simulink model "ROSCO_vs_ESC"  (R2025b)
settings: Solver=VariableStepAuto  StartTime=0.0  StopTime=4000  RelTol=1e-3
undefined symbols (not defined in the file): J, K_tau, ki_tau, kp_tau, lambda_opt, Ng, omega_g_min, omega_g_rated, R, tau_g_rated
libraries: simulink x1
settings Model: Creator=Administrator  LastModifiedBy=Administrator
settings DataIOCC: ReturnWorkspaceOutputs=off

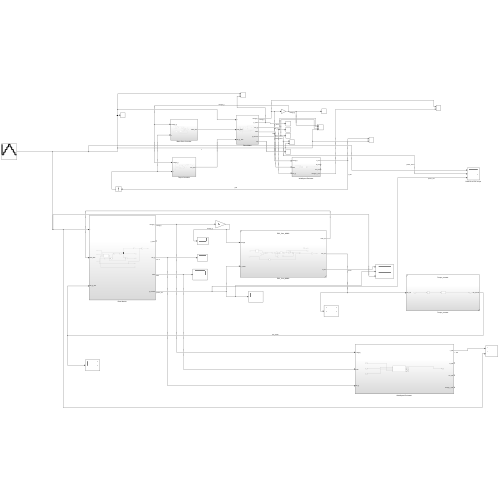
[thumbnail: Simulink's stored preview of the top-level diagram]
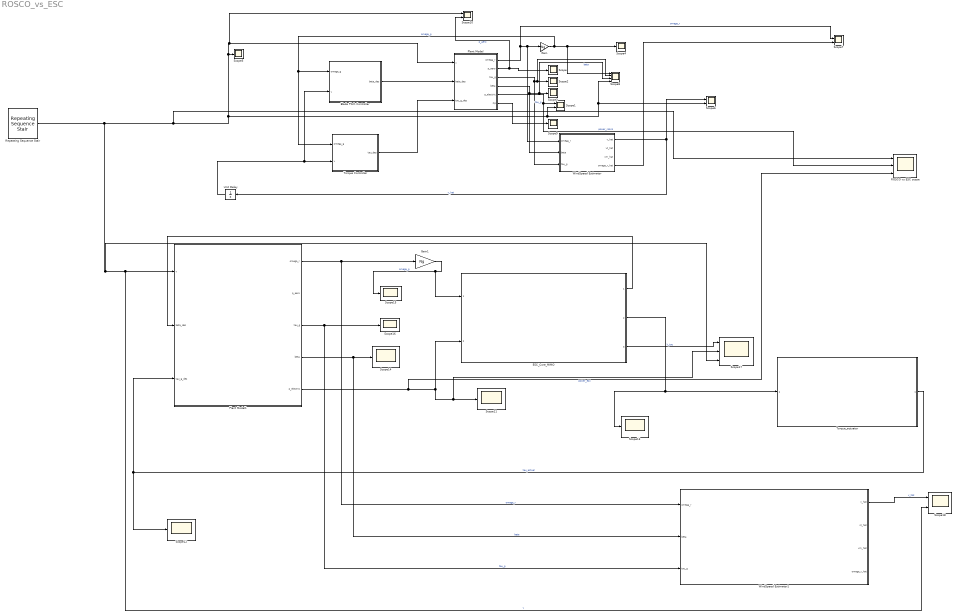
== system ROSCO_vs_ESC ==
  Blade Pitch Controller : Subsystem
  ESC_Core_MIMO : Subsystem  ReferencedSubsystem=ESC_Core_MIMO
  Gain : Gain  Gain=Ng
  Gain1 : Gain  Gain=Ng
  Plant Model : Subsystem
  Plant Model1 : Subsystem
  ROSCO vs ESC scope : Scope  NumInputPorts=3
      settings: ActiveDisplayYMinimum=5.5  ActiveDisplayYMaximum=10.5  DataLoggingVariableName=velData
  Repeating Sequence Stair : simulink/Sources/Repeating Sequence Stair  OutValues=[6 7 8 9 10 9 8 7 6]  tsamp=400  OutMin=[]  OutMax=[]  OutDataTypeStr=double  OutputDataTypeScalingMode=double  OutDataType=fixdt(0,8)  ConRadixGroup=Best Precision: Vector-wise  OutScaling=2^-12
  Scope{,2..5,9,11..16} (12 alike) : Scope
      Scope settings: ActiveDisplayYMinimum=-2.4283893779933713E+6  ActiveDisplayYMaximum=1.2562737180596253E+7  DataLoggingVariableName=ScopeData17
      Scope11 settings: ActiveDisplayYMinimum=-206726.94893270766  ActiveDisplayYMaximum=1.8605425403943695E+6  DataLoggingVariableName=ScopeData24
      Scope12 settings: ActiveDisplayYMinimum=25883.443415286834  ActiveDisplayYMaximum=45883.443415286834  DataLoggingVariableName=ScopeData25
      Scope13 settings: ActiveDisplayYMinimum=-6959.4378100502436  ActiveDisplayYMaximum=51916.667459968325  DataLoggingVariableName=ScopeData26
      Scope14 settings: ActiveDisplayYMinimum=-0.028992577845199295  ActiveDisplayYMaximum=0.2609332006067937  DataLoggingVariableName=ScopeData27
      Scope15 settings: ActiveDisplayYMinimum=5.9360506198945675  ActiveDisplayYMaximum=140.57554442094894  DataLoggingVariableName=ScopeData28
      Scope16 settings: ActiveDisplayYMinimum=-1  ActiveDisplayYMaximum=1  DataLoggingVariableName=ScopeData29
      Scope2 settings: ActiveDisplayYMinimum=-1  ActiveDisplayYMaximum=1  DataLoggingVariableName=ScopeData19
      Scope3 settings: ActiveDisplayYMinimum=-5.1281576222926013  ActiveDisplayYMaximum=18.391881826207097  DataLoggingVariableName=ScopeData4
      Scope4 settings: ActiveDisplayYMinimum=-16.100769807351526  ActiveDisplayYMaximum=150.23183145512027  DataLoggingVariableName=ScopeData5
      Scope5 settings: ActiveDisplayYMinimum=-1.9549334631606692  ActiveDisplayYMaximum=17.594401168446026  DataLoggingVariableName=ScopeData20
      Scope9 settings: ActiveDisplayYMinimum=-1  ActiveDisplayYMaximum=1  DataLoggingVariableName=ScopeData8
  Scope{1,6..7,10,18} (5 alike) : Scope  NumInputPorts=2
      Scope1 settings: ActiveDisplayYMinimum=1  ActiveDisplayYMaximum=21  DataLoggingVariableName=ScopeData18
      Scope10 settings: ActiveDisplayYMinimum=-0.49921784144822823  ActiveDisplayYMaximum=25.750782158551765  DataLoggingVariableName=ScopeData16
      Scope18 settings: ActiveDisplayYMinimum=-1.2495467804496814  ActiveDisplayYMaximum=11.245921024047135  DataLoggingVariableName=ScopeData31
      Scope6 settings: ActiveDisplayYMinimum=-1  ActiveDisplayYMaximum=1  DataLoggingVariableName=ScopeData21
      Scope7 settings: ActiveDisplayYMinimum=0.05875  ActiveDisplayYMaximum=1.47128  DataLoggingVariableName=ScopeData22
  Scope17 : Scope  NumInputPorts=3
      settings: ActiveDisplayYMinimum=2.97179268816189  ActiveDisplayYMaximum=7.2893156949682956  DataLoggingVariableName=ScopeData30
  Scope8 : Scope  NumInputPorts=4
      settings: ActiveDisplayYMinimum=5.68642269301175  ActiveDisplayYMaximum=142.8221957628943  DataLoggingVariableName=ScopeData23
  Torque Controller : Subsystem
  Torque_actuator : Subsystem  ReferencedSubsystem=Torque_actuator
  Unit Delay : UnitDelay  SampleTime=0.01  HasFrameUpgradeWarning=on
  WindSpeed Estimator : Subsystem
  WindSpeed Estimator1 : Subsystem
  wires:
  Plant Model/3(tau_g) -> Scope8/2, Scope2/1, WindSpeed Estimator/3(tau_g)  "tau_g"
  WindSpeed Estimator/4(omega_r_hat) -> Scope7/2
  Repeating Sequence Stair/1 -> Scope17/3, Scope18/2, Plant Model1/1(v), ROSCO vs ESC scope/1, Scope5/1, Scope10/1, Plant Model/1(v), Scope1/2, Scope8/4, Scope6/2  "v"
  WindSpeed Estimator/1(v_hat) -> Unit Delay/1, Scope6/1  "v_hat"
  Unit Delay/1 -> Blade Pitch Controller/2(v), Torque Controller/2(v)
  Torque Controller/1(tau_des) -> Plant Model/3(tau_g_des)
  Plant Model/6(Cp) -> Scope9/1
  Plant Model/2(p_aero) -> Scope10/2, Scope/1  "p_aero"
  Blade Pitch Controller/1(beta_des) -> Plant Model/2(beta_des)
  Gain/1 -> Blade Pitch Controller/1(omega_g), Torque Controller/1(omega_g), Scope8/1, Scope4/1  "omega_g"
  Plant Model/1(omega_r) -> WindSpeed Estimator/1(omega_r), Gain/1, Scope7/1  "omega_r"
  Plant Model/4(beta) -> Scope8/3, Scope3/1, WindSpeed Estimator/2(beta)  "beta"
  Plant Model/5(p_electric) -> ROSCO vs ESC scope/2, Scope1/1  "power_rosco"
  Plant Model1/3(tau_g) -> WindSpeed Estimator1/3(tau_g), Scope16/1  "tau_g"
  Torque_actuator/1 -> Scope12/1, Plant Model1/3(tau_g_des)  "tau_actual"
  Plant Model1/1(omega_r) -> WindSpeed Estimator1/1(omega_r), Gain1/1  "omega_r"
  ESC_Core_MIMO/3 -> Scope17/1  "k_tau"
  Plant Model1/5(p_electric) -> ROSCO vs ESC scope/3, Scope17/2, Scope11/1, ESC_Core_MIMO/2  "power_esc"
  ESC_Core_MIMO/1 -> Plant Model1/2(beta_des)
  Plant Model1/4(beta) -> WindSpeed Estimator1/2(beta), Scope14/1  "beta"
  WindSpeed Estimator1/1(v_hat) -> Scope18/1  "v_hat"
  Gain1/1 -> Scope15/1, ESC_Core_MIMO/1  "omega_g"
  ESC_Core_MIMO/2 -> Torque_actuator/1, Scope13/1

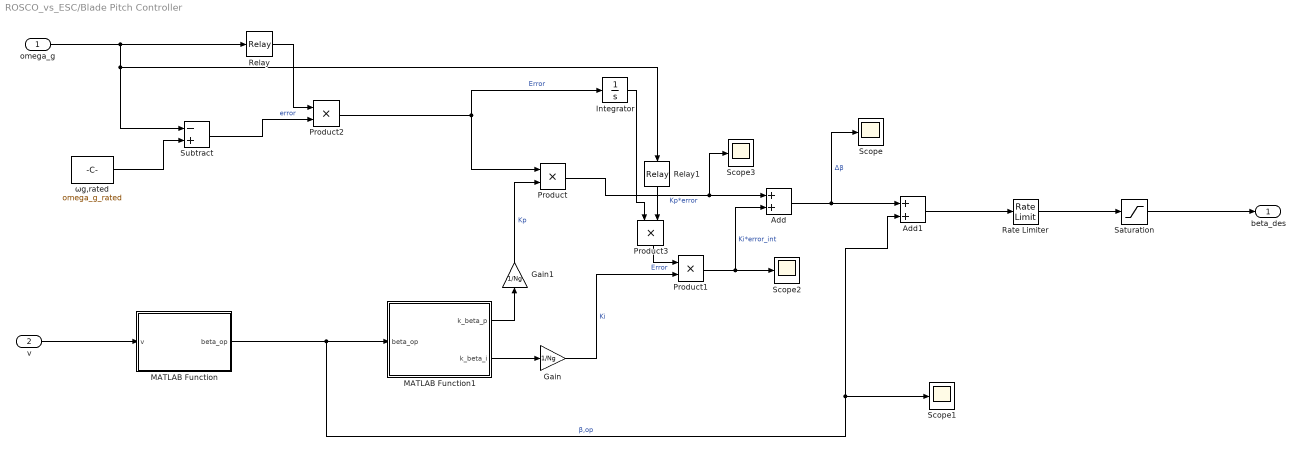
== system ROSCO_vs_ESC/Blade Pitch Controller ==
  omega_g : Inport
  v : Inport  Port=2
  Add : Sum
  Add1 : Sum
  Gain : Gain  Gain=1/Ng
  Gain1 : Gain  Gain=1/Ng
  Integrator : Integrator
  MATLAB Function : MATLAB Function  TreatAsAtomicUnit=on
  MATLAB Function1 : MATLAB Function  TreatAsAtomicUnit=on
  Product{,1..3} (4 alike) : Product
  Rate Limiter : RateLimiter  RisingSlewLimit=8  FallingSlewLimit=-8  SampleTimeMode=inherited
  Relay : Relay  OnSwitchValue=123.91  OffSwitchValue=121.91
  Relay1 : Relay  OnSwitchValue=123.91  OffSwitchValue=121.91
  Saturation : Saturate  UpperLimit=25  LowerLimit=0
  Scope{,1..3} (4 alike) : Scope
      Scope settings: ActiveDisplayYMinimum=-1  ActiveDisplayYMaximum=1  DataLoggingVariableName=ScopeData6
      Scope1 settings: ActiveDisplayYMinimum=-1  ActiveDisplayYMaximum=1  DataLoggingVariableName=ScopeData7
      Scope2 settings: ActiveDisplayYMinimum=-1  ActiveDisplayYMaximum=1  DataLoggingVariableName=ScopeData14
      Scope3 settings: ActiveDisplayYMinimum=-1  ActiveDisplayYMaximum=1  DataLoggingVariableName=ScopeData15
  Subtract : Sum  Inputs=-+
  ωg,rated : Constant  Value=omega_g_rated
  beta_des : Outport
  wires:
  Product1/1 -> Scope2/1, Add/2  "Ki*error_int"
  Add/1 -> Scope/1, Add1/1  "Δβ"
  MATLAB Function1/2(k_beta_i) -> Gain/1
  MATLAB Function/1(beta_op) -> Scope1/1, Add1/2, MATLAB Function1/1(beta_op)  "β,op"
  Product/1 -> Scope3/1, Add/1  "Kp*error"
  v/1 -> MATLAB Function/1(v)
  MATLAB Function1/1(k_beta_p) -> Gain1/1
  omega_g/1 -> Subtract/1, Relay1/1, Relay/1
  ωg,rated/1 -> Subtract/2
  Gain/1 -> Product1/2  "Ki"
  Gain1/1 -> Product/2  "Kp"
  Relay/1 -> Product2/1
  Subtract/1 -> Product2/2  "error"
  Product2/1 -> Integrator/1, Product/1  "Error"
  Rate Limiter/1 -> Saturation/1
  Saturation/1 -> beta_des/1
  Add1/1 -> Rate Limiter/1
  Relay1/1 -> Product3/2
  Integrator/1 -> Product3/1
  Product3/1 -> Product1/1  "Error"

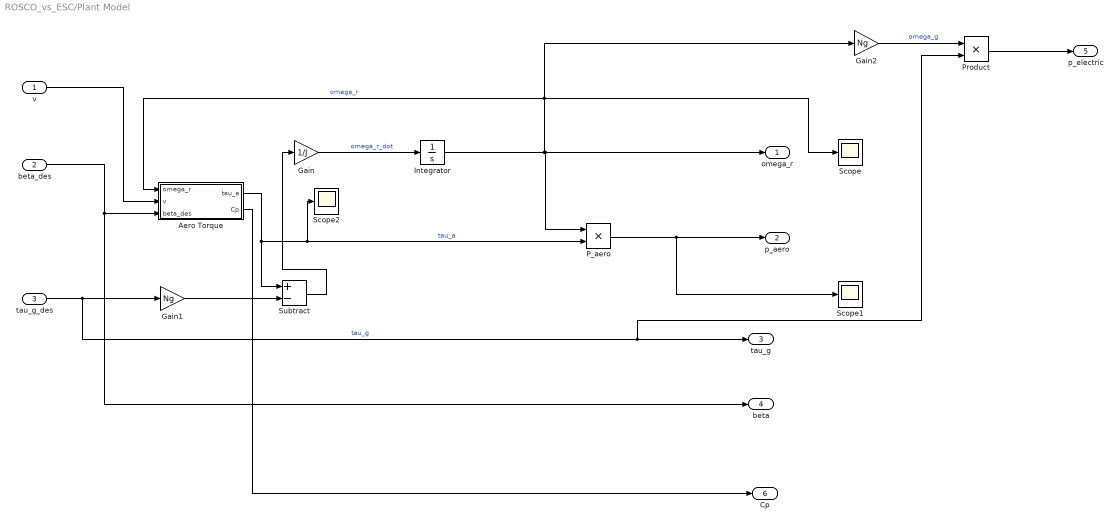
== system ROSCO_vs_ESC/Plant Model ==
  v : Inport
  beta_des : Inport  Port=2
  tau_g_des : Inport  Port=3
  Aero Torque : Subsystem
  Gain : Gain  Gain=1/J
  Gain1 : Gain  Gain=Ng
  Gain2 : Gain  Gain=Ng
  Integrator : Integrator  InitialCondition=0.2
  P_aero : Product
  Product : Product
  Scope : Scope
      settings: ActiveDisplayYMinimum=0.04836  ActiveDisplayYMaximum=1.56476
  Scope1 : Scope
      settings: ActiveDisplayYMinimum=2.19667122099E+6  ActiveDisplayYMaximum=6.12528052336E+6
  Scope2 : Scope
      settings: ActiveDisplayYMinimum=-1.02218292866E+6  ActiveDisplayYMaximum=9.19964635791E+6
  Subtract : Sum  Inputs=+-
  omega_r : Outport
  p_aero : Outport  Port=2
  tau_g : Outport  Port=3
  beta : Outport  Port=4
  p_electric : Outport  Port=5
  Cp : Outport  Port=6
  wires:
  v/1 -> Aero Torque/2(v)
  Aero Torque/1(tau_a) -> Scope2/1, P_aero/2, Subtract/1  "tau_a"
  Gain1/1 -> Subtract/2
  Integrator/1 -> Gain2/1, Scope/1, Aero Torque/1(omega_r), omega_r/1, P_aero/1  "omega_r"
  beta_des/1 -> beta/1, Aero Torque/3(beta_des)
  P_aero/1 -> p_aero/1, Scope1/1
  Subtract/1 -> Gain/1
  Gain/1 -> Integrator/1  "omega_r_dot"
  tau_g_des/1 -> Product/2, tau_g/1, Gain1/1  "tau_g"
  Gain2/1 -> Product/1  "omega_g"
  Product/1 -> p_electric/1
  Aero Torque/2(Cp) -> Cp/1

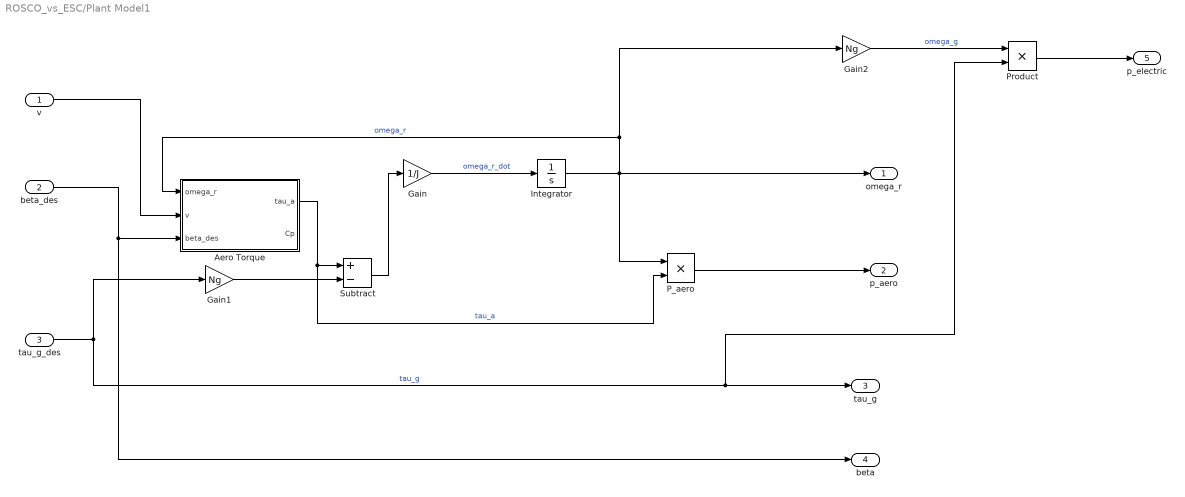
== system ROSCO_vs_ESC/Plant Model1 ==
  v : Inport
  beta_des : Inport  Port=2
  tau_g_des : Inport  Port=3
  Aero Torque : Subsystem
  Gain : Gain  Gain=1/J
  Gain1 : Gain  Gain=Ng
  Gain2 : Gain  Gain=Ng
  Integrator : Integrator  InitialCondition=0.2
  P_aero : Product
  Product : Product
  Subtract : Sum  Inputs=+-
  omega_r : Outport
  p_aero : Outport  Port=2
  tau_g : Outport  Port=3
  beta : Outport  Port=4
  p_electric : Outport  Port=5
  wires:
  v/1 -> Aero Torque/2(v)
  Aero Torque/1(tau_a) -> P_aero/2, Subtract/1  "tau_a"
  Gain1/1 -> Subtract/2
  Integrator/1 -> Gain2/1, Aero Torque/1(omega_r), omega_r/1, P_aero/1  "omega_r"
  beta_des/1 -> beta/1, Aero Torque/3(beta_des)
  P_aero/1 -> p_aero/1
  Subtract/1 -> Gain/1
  Gain/1 -> Integrator/1  "omega_r_dot"
  tau_g_des/1 -> Product/2, tau_g/1, Gain1/1  "tau_g"
  Gain2/1 -> Product/1  "omega_g"
  Product/1 -> p_electric/1

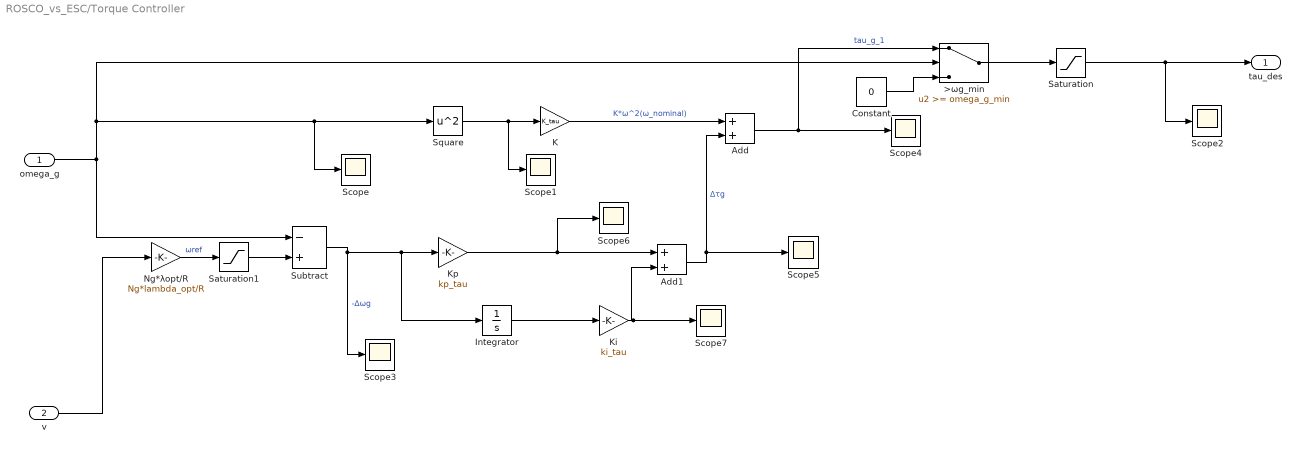
== system ROSCO_vs_ESC/Torque Controller ==
  omega_g : Inport
  v : Inport  Port=2
  >ωg_min : Switch  Threshold=omega_g_min  ZeroCross=off  SaturateOnIntegerOverflow=off  InputSameDT=off
  Add : Sum
  Add1 : Sum
  Constant : Constant  Value=0
  Integrator : Integrator
  K : Gain  Gain=K_tau
  Ki : Gain  Gain=ki_tau
  Kp : Gain  Gain=kp_tau
  Ng*λopt/R : Gain  Gain=Ng*lambda_opt/R
  Saturation : Saturate  UpperLimit=tau_g_rated  LowerLimit=0
  Saturation1 : Saturate  UpperLimit=omega_g_rated  LowerLimit=omega_g_min
  Scope{,1..7} (8 alike) : Scope
      Scope settings: ActiveDisplayYMinimum=4.69097  ActiveDisplayYMaximum=151.78129
      Scope1 settings: ActiveDisplayYMinimum=-1655.7009946609019  ActiveDisplayYMaximum=18664.908951948124  DataLoggingVariableName=ScopeData2
      Scope2 settings: ActiveDisplayYMinimum=-4328.10328  ActiveDisplayYMaximum=38952.92956  DataLoggingVariableName=ScopeData3
      Scope3 settings: ActiveDisplayYMinimum=-28.87171  ActiveDisplayYMaximum=118.21861  DataLoggingVariableName=ScopeData10
      Scope4 settings: ActiveDisplayYMinimum=-75728.80233  ActiveDisplayYMaximum=46886.34056  DataLoggingVariableName=ScopeData9
      Scope5 settings: ActiveDisplayYMinimum=-72200.05859  ActiveDisplayYMaximum=6234.76791  DataLoggingVariableName=ScopeData11
      Scope6 settings: ActiveDisplayYMinimum=-73501.84527  ActiveDisplayYMaximum=17950.84803  DataLoggingVariableName=ScopeData12
      Scope7 settings: ActiveDisplayYMinimum=-1  ActiveDisplayYMaximum=1  DataLoggingVariableName=ScopeData13
  Square : Math  Operator=square
  Subtract : Sum  Inputs=-+
  tau_des : Outport
  wires:
  Ki/1 -> Add1/2, Scope7/1
  Add/1 -> Scope4/1, >ωg_min/1  "tau_g_1"
  omega_g/1 -> Subtract/1, >ωg_min/2, Scope/1, Square/1
  Square/1 -> Scope1/1, K/1
  Ng*λopt/R/1 -> Saturation1/1  "ωref"
  v/1 -> Ng*λopt/R/1
  Subtract/1 -> Scope3/1, Integrator/1, Kp/1  "-Δωg"
  Constant/1 -> >ωg_min/3
  K/1 -> Add/1  "K*ω^2(ω_nominal)"
  Add1/1 -> Add/2, Scope5/1  "Δτg"
  >ωg_min/1 -> Saturation/1
  Saturation/1 -> Scope2/1, tau_des/1
  Saturation1/1 -> Subtract/2
  Kp/1 -> Scope6/1, Add1/1
  Integrator/1 -> Ki/1

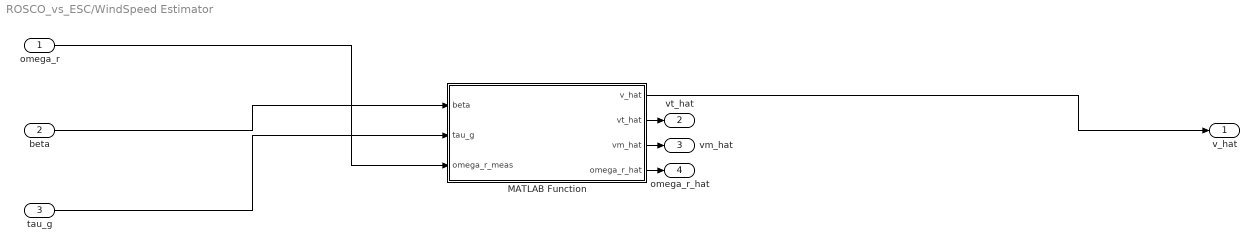
== system ROSCO_vs_ESC/WindSpeed Estimator ==
  omega_r : Inport
  beta : Inport  Port=2
  tau_g : Inport  Port=3
  MATLAB Function : MATLAB Function  TreatAsAtomicUnit=on  SystemSampleTime=0.01
  v_hat : Outport
  vt_hat : Outport  Port=2
  vm_hat : Outport  Port=3
  omega_r_hat : Outport  Port=4
  wires:
  MATLAB Function/3(vm_hat) -> vm_hat/1
  tau_g/1 -> MATLAB Function/2(tau_g)
  MATLAB Function/4(omega_r_hat) -> omega_r_hat/1
  MATLAB Function/1(v_hat) -> v_hat/1
  beta/1 -> MATLAB Function/1(beta)
  omega_r/1 -> MATLAB Function/3(omega_r_meas)
  MATLAB Function/2(vt_hat) -> vt_hat/1

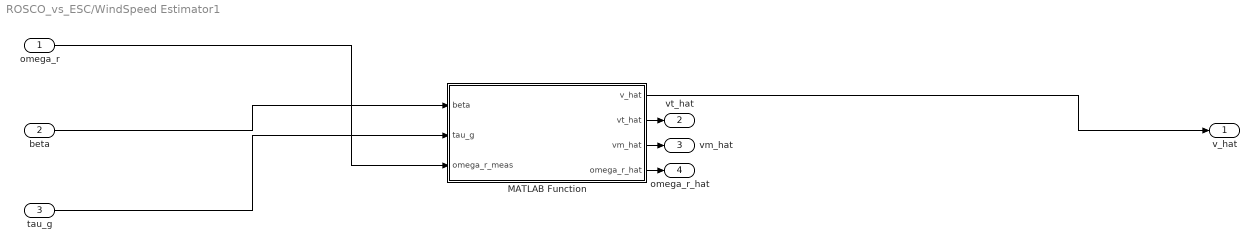
== system ROSCO_vs_ESC/WindSpeed Estimator1 ==
  omega_r : Inport
  beta : Inport  Port=2
  tau_g : Inport  Port=3
  MATLAB Function : MATLAB Function  TreatAsAtomicUnit=on  SystemSampleTime=0.01
  v_hat : Outport
  vt_hat : Outport  Port=2
  vm_hat : Outport  Port=3
  omega_r_hat : Outport  Port=4
  wires:
  MATLAB Function/3(vm_hat) -> vm_hat/1
  tau_g/1 -> MATLAB Function/2(tau_g)
  MATLAB Function/4(omega_r_hat) -> omega_r_hat/1
  MATLAB Function/1(v_hat) -> v_hat/1
  beta/1 -> MATLAB Function/1(beta)
  omega_r/1 -> MATLAB Function/3(omega_r_meas)
  MATLAB Function/2(vt_hat) -> vt_hat/1

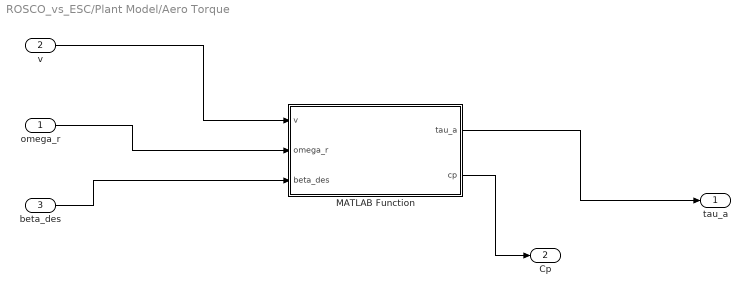
== system ROSCO_vs_ESC/Plant Model/Aero Torque ==
  omega_r : Inport
  v : Inport  Port=2
  beta_des : Inport  Port=3
  MATLAB Function : MATLAB Function  TreatAsAtomicUnit=on
  tau_a : Outport
  Cp : Outport  Port=2
  wires:
  v/1 -> MATLAB Function/1(v)
  omega_r/1 -> MATLAB Function/2(omega_r)
  beta_des/1 -> MATLAB Function/3(beta_des)
  MATLAB Function/1(tau_a) -> tau_a/1
  MATLAB Function/2(cp) -> Cp/1

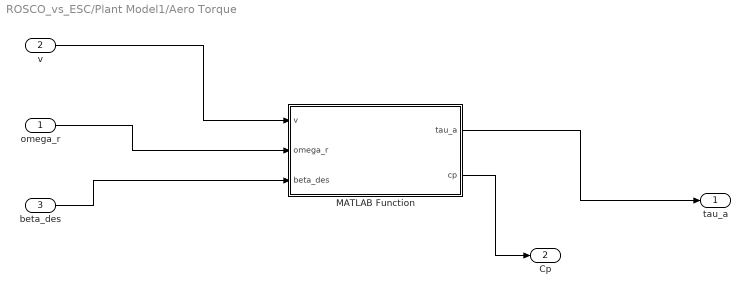
== system ROSCO_vs_ESC/Plant Model1/Aero Torque ==
  omega_r : Inport
  v : Inport  Port=2
  beta_des : Inport  Port=3
  MATLAB Function : MATLAB Function  TreatAsAtomicUnit=on
  tau_a : Outport
  Cp : Outport  Port=2
  wires:
  v/1 -> MATLAB Function/1(v)
  omega_r/1 -> MATLAB Function/2(omega_r)
  beta_des/1 -> MATLAB Function/3(beta_des)
  MATLAB Function/1(tau_a) -> tau_a/1
  MATLAB Function/2(cp) -> Cp/1

== matlab function ROSCO_vs_ESC/Blade Pitch Controller/MATLAB Function ==
  data: v input; beta_op output
function beta_op = beta_op_from_v(v)

    v_table = [ ...
        11.4  12.4  13.4  14.4  15.4  ...
        16.4  17.4  18.4  19.4  20.4  ...
        21.4  22.4  23.4  24.4  25.4 ];

    beta_table = [ ...
         0.00    6.80   11.25   15.00   17.30 ...
        19.65   21.85   23.90   25.00   25.00 ...
        25.00   25.00   25.00   25.00   25.00 ];
    
    if v <= v_table(1)
        beta_op = beta_table(1);
    elseif v >= v_table(end)
        beta_op = beta_table(end);
    else
        beta_op = interp1(v_table, beta_table, v, 'linear');
    end
end

== matlab function ROSCO_vs_ESC/Plant Model/Aero Torque/MATLAB Function ==
  data: v input; tau_a output; omega_r input; beta_des input; cp output
function [tau_a,cp] = aero_torque(v, omega_r, beta_des)

    rho = 1.225;      
    R   = 63;         
    A   = pi*R^2; 
    lambda = omega_r * R / v;
    omega_eps = 0.1;   % rad/s
    v_eps     = 0.1;   % m/s
    
    omega_eff = omega_r;
    if abs(omega_eff) < omega_eps
        omega_eff = omega_eps * sign(omega_eff + 1e-6);
    end

    
    v_eff = v;
    if abs(v_eff) < v_eps
        v_eff = v_eps;
    end
    

    
    lambda_vec = [0 4 6 8 10 12 14];
beta_vec   = [0 5 10 15 20 25];

Cp_table = [
    0.000 0.299 0.436 0.389 0.248 0.073 0.000;
    0.000 0.249 0.347 0.338 0.274 0.187 0.095;
    0.000 0.247 0.282 0.222 0.120 0.005 0.000;
    0.000 0.225 0.198 0.091 0.000 0.000 0.000;
    0.000 0.182 0.096 0.000 0.000 0.000 0.000;
    0.000 0.119 0.000 0.000 0.000 0.000 0.000
];

   lambda = min(max(lambda, lambda_vec(1)), lambda_vec(end));
   beta_des   = min(max(beta_des,   beta_vec(1)),   beta_vec(end)); 
   cp = interp2(lambda_vec, beta_vec, Cp_table, ...
                 lambda, beta_des, 'linear');
    tau_a = 0.5 * rho * A * (v_eff^3 / omega_eff) * cp;
end

== matlab function ROSCO_vs_ESC/Blade Pitch Controller/MATLAB Function1 ==
  data: beta_op input; k_beta_p output; k_beta_i output
function [k_beta_p, k_beta_i] = AB_from_beta(beta_op)

    beta_table = [ ...
         0.000000  6.800000  11.200000  15.000000  ...
        17.300000  19.600000  21.800000  23.900000 ];

    A_table = [ ...
        -0.104264  -0.094339  -0.059128  -0.101610  ...
        -0.139651  -0.187221  -0.228149  -0.270746 ];

    B_table = [ ...
        -0.280148  -0.435376  -0.596426  -0.708989  ...
        -0.853208  -0.907132  -1.148247  -1.280977 ];
    

   
    if beta_op <= beta_table(1)
        A_out = A_table(1);
        B_out = B_table(1);
    elseif beta_op >= beta_table(end)
        A_out = A_table(end);
        B_out = B_table(end);
    else
        
        A_out = interp1(beta_table, A_table, beta_op, 'linear');
        B_out = interp1(beta_table, B_table, beta_op, 'linear');
    end
    damp_beta_des = 0.7;
    omega_beta_des = 0.7;
    k_beta_p = (2*omega_beta_des*damp_beta_des+A_out)/B_out;
    k_beta_i = omega_beta_des^2/B_out;
end

== matlab function ROSCO_vs_ESC/WindSpeed Estimator/MATLAB Function ==
  data: beta input; tau_g input; v_hat output; omega_r_meas input; vt_hat output; vm_hat output; omega_r_hat output
function [v_hat, vt_hat, vm_hat, omega_r_hat] = WSE_EKF(beta, tau_g, omega_r_meas)
%% ---------- constants  ----------
Ts  = 0.01;        
Ng  = 97;          % gearbox ratio
J   = 3.87e7;      % rotor inertia (rotor side)
R   = 63;          % rotor radius
rho = 1.225;
Arot = pi*R^2;

L  = 6.0 * R;      % length scale
Ti = 0.18;         % turbulence intensity
Rm = 0.02;         % meas noise var (omega_r)

q_omega = 1e-5;
q_vm    = (2.0^2)/600.0;

OM_MIN = 0.1;
V_MIN  = 0.1;

%% ---------- persistent states ----------
persistent x_hat P K_prev initFlag
if isempty(initFlag)
    initFlag = uint8(0);
    x_hat = zeros(3,1);
    P = eye(3);
    K_prev = zeros(3,1);
end

if initFlag == 0
    x_hat(1) = omega_r_meas;  % omega_r0
    x_hat(2) = 0.0;           % vt0
    x_hat(3) = 8.0;           % vm0 
    P = diag([0.01, 0.01, 1.0]);
    K_prev = zeros(3,1);
    initFlag = uint8(1);
end

%% ---------- unpack ----------
omega_r = max(x_hat(1), OM_MIN);
vt      = x_hat(2);
vm      = x_hat(3);

v_est = max(vt + vm, V_MIN);

%% ---------- Cp lookup table  ----------
lambda_vec = [0 4 6 8 10 12 14];
beta_vec   = [0 5 10 15 20 25];

Cp_table = [ ...
0.000 0.299 0.436 0.389 0.248 0.073 0.000;  % beta=0
0.000 0.249 0.347 0.338 0.274 0.187 0.095;  % beta=5
0.000 0.247 0.282 0.222 0.120 0.005 0.000;  % beta=10
0.000 0.225 0.198 0.091 0.000 0.000 0.000;  % beta=15
0.000 0.182 0.096 0.000 0.000 0.000 0.000;  % beta=20
0.000 0.119 0.000 0.000 0.000 0.000 0.000]; % beta=25

%% ---------- helper: aero torque at current x_hat ----------
lambda = omega_r * R / v_est;
lambda = min(max(lambda, lambda_vec(1)), lambda_vec(end));
beta_c = min(max(beta,   beta_vec(1)),   beta_vec(end));

Cp = interp2(lambda_vec, beta_vec, Cp_table, lambda, beta_c, 'linear');

P_a = 0.5 * rho * Arot * Cp * (v_est^3);
tau_a = P_a / omega_r;

%% ---------- continuous dynamics f(x,u) ----------
omega_r_dot = (tau_a - Ng*tau_g)/J;
a_vm = (pi*max(vm, V_MIN))/(2.0*L);
vt_dot = -a_vm*vt;
vm_dot = 0.0;

f = [omega_r_dot; vt_dot; vm_dot];

%% ---------- prediction  ----------
x_pred = x_hat + Ts*f;

%% ---------- Jacobian F via finite difference ----------
epsFD = 1e-4;
F = zeros(3,3);

for i = 1:3
    dx = zeros(3,1); dx(i) = epsFD;
    x_p = x_hat + dx;

    om_p = max(x_p(1), OM_MIN);
    vt_p = x_p(2);
    vm_p = x_p(3);
    v_p  = max(vt_p + vm_p, V_MIN);

    lambda_p = om_p * R / v_p;
    lambda_p = min(max(lambda_p, lambda_vec(1)), lambda_vec(end));
    beta_p   = min(max(beta,      beta_vec(1)),   beta_vec(end));

    Cp_p = interp2(lambda_vec, beta_vec, Cp_table, lambda_p, beta_p, 'linear');
    P_a_p = 0.5 * rho * Arot * Cp_p * (v_p^3);
    tau_a_p = P_a_p / om_p;

    om_dot_p = (tau_a_p - Ng*tau_g)/J;
    a_vm_p   = (pi*max(vm_p, V_MIN))/(2.0*L);
    vt_dot_p = -a_vm_p*vt_p;
    vm_dot_p = 0.0;

    f_p = [om_dot_p; vt_dot_p; vm_dot_p];
    F(:,i) = (f_p - f)/epsFD;
end

%% ---------- Q  ----------
vm_for_Q = max(vm, 0.1);
Q = zeros(3,3);
Q(1,1) = q_omega;
Q(2,2) = pi*(vm_for_Q^3)*(Ti^2)/L;
Q(3,3) = q_vm;

%% ---------- covariance prediction  ----------
Pdot   = F*P + P*F' + Q - (K_prev*Rm*K_prev');
P_pred = P + Ts*Pdot;

%% ---------- measurement update ----------
H = [1 0 0];
y = omega_r_meas;

innov = y - x_pred(1);
S = H*P_pred*H' + Rm;
K = (P_pred*H')/S;

x_upd = x_pred + K*innov;
P_upd = (eye(3) - K*H) * P_pred;

x_hat  = x_upd;
P      = P_upd;
K_prev = K;

%% ---------- outputs ----------
omega_r_hat = x_hat(1);
vt_hat      = x_hat(2);
vm_hat      = x_hat(3);
v_hat       = vt_hat + vm_hat;
end

== matlab function ROSCO_vs_ESC/Plant Model1/Aero Torque/MATLAB Function ==
  data: v input; tau_a output; omega_r input; beta_des input; cp output
function [tau_a,cp] = aero_torque(v, omega_r, beta_des)

    rho = 1.225;      
    R   = 63;         
    A   = pi*R^2; 
    lambda = omega_r * R / v;
    omega_eps = 0.1;   % rad/s
    v_eps     = 0.1;   % m/s
    
    omega_eff = omega_r;
    if abs(omega_eff) < omega_eps
        omega_eff = omega_eps * sign(omega_eff + 1e-6);
    end

    
    v_eff = v;
    if abs(v_eff) < v_eps
        v_eff = v_eps;
    end
    

    % 气动力矩公式：tau_a = 0.5 * rho * A * (v^3 / omega_r) * Cp
    lambda_vec = [0 4 6 8 10 12 14];
beta_vec   = [0 5 10 15 20 25];

Cp_table = [
    0.000 0.299 0.436 0.389 0.248 0.073 0.000;
    0.000 0.249 0.347 0.338 0.274 0.187 0.095;
    0.000 0.247 0.282 0.222 0.120 0.005 0.000;
    0.000 0.225 0.198 0.091 0.000 0.000 0.000;
    0.000 0.182 0.096 0.000 0.000 0.000 0.000;
    0.000 0.119 0.000 0.000 0.000 0.000 0.000
];

   lambda = min(max(lambda, lambda_vec(1)), lambda_vec(end));
   beta_des   = min(max(beta_des,   beta_vec(1)),   beta_vec(end)); 
   cp = interp2(lambda_vec, beta_vec, Cp_table, ...
                 lambda, beta_des, 'linear');
    tau_a = 0.5 * rho * A * (v_eff^3 / omega_eff) * cp;
end

== matlab function ROSCO_vs_ESC/WindSpeed Estimator1/MATLAB Function ==
  data: beta input; tau_g input; v_hat output; omega_r_meas input; vt_hat output; vm_hat output; omega_r_hat output
function [v_hat, vt_hat, vm_hat, omega_r_hat] = WSE_EKF(beta, tau_g, omega_r_meas)
%% ---------- constants  ----------
Ts  = 0.01;        
Ng  = 97;          % gearbox ratio
J   = 3.87e7;      % rotor inertia (rotor side)
R   = 63;          % rotor radius
rho = 1.225;
Arot = pi*R^2;

L  = 6.0 * R;      % length scale
Ti = 0.18;         % turbulence intensity
Rm = 0.02;         % meas noise var (omega_r)

q_omega = 1e-5;
q_vm    = (2.0^2)/600.0;

OM_MIN = 0.1;
V_MIN  = 0.1;

%% ---------- persistent states ----------
persistent x_hat P K_prev initFlag
if isempty(initFlag)
    initFlag = uint8(0);
    x_hat = zeros(3,1);
    P = eye(3);
    K_prev = zeros(3,1);
end

if initFlag == 0
    x_hat(1) = omega_r_meas;  % omega_r0
    x_hat(2) = 0.0;           % vt0
    x_hat(3) = 8.0;           % vm0 
    P = diag([0.01, 0.01, 1.0]);
    K_prev = zeros(3,1);
    initFlag = uint8(1);
end

%% ---------- unpack ----------
omega_r = max(x_hat(1), OM_MIN);
vt      = x_hat(2);
vm      = x_hat(3);

v_est = max(vt + vm, V_MIN);

%% ---------- Cp lookup table ) ----------
lambda_vec = [0 4 6 8 10 12 14];
beta_vec   = [0 5 10 15 20 25];

Cp_table = [ ...
0.000 0.299 0.436 0.389 0.248 0.073 0.000;  % beta=0
0.000 0.249 0.347 0.338 0.274 0.187 0.095;  % beta=5
0.000 0.247 0.282 0.222 0.120 0.005 0.000;  % beta=10
0.000 0.225 0.198 0.091 0.000 0.000 0.000;  % beta=15
0.000 0.182 0.096 0.000 0.000 0.000 0.000;  % beta=20
0.000 0.119 0.000 0.000 0.000 0.000 0.000]; % beta=25

%% ---------- helper: aero torque at current x_hat ----------
lambda = omega_r * R / v_est;
lambda = min(max(lambda, lambda_vec(1)), lambda_vec(end));
beta_c = min(max(beta,   beta_vec(1)),   beta_vec(end));

Cp = interp2(lambda_vec, beta_vec, Cp_table, lambda, beta_c, 'linear');

P_a = 0.5 * rho * Arot * Cp * (v_est^3);
tau_a = P_a / omega_r;

%% ---------- continuous dynamics f(x,u) ----------
omega_r_dot = (tau_a - Ng*tau_g)/J;
a_vm = (pi*max(vm, V_MIN))/(2.0*L);
vt_dot = -a_vm*vt;
vm_dot = 0.0;

f = [omega_r_dot; vt_dot; vm_dot];

%% ---------- prediction  ----------
x_pred = x_hat + Ts*f;

%% ---------- Jacobian F via finite difference ----------
epsFD = 1e-4;
F = zeros(3,3);

for i = 1:3
    dx = zeros(3,1); dx(i) = epsFD;
    x_p = x_hat + dx;

    om_p = max(x_p(1), OM_MIN);
    vt_p = x_p(2);
    vm_p = x_p(3);
    v_p  = max(vt_p + vm_p, V_MIN);

    lambda_p = om_p * R / v_p;
    lambda_p = min(max(lambda_p, lambda_vec(1)), lambda_vec(end));
    beta_p   = min(max(beta,      beta_vec(1)),   beta_vec(end));

    Cp_p = interp2(lambda_vec, beta_vec, Cp_table, lambda_p, beta_p, 'linear');
    P_a_p = 0.5 * rho * Arot * Cp_p * (v_p^3);
    tau_a_p = P_a_p / om_p;

    om_dot_p = (tau_a_p - Ng*tau_g)/J;
    a_vm_p   = (pi*max(vm_p, V_MIN))/(2.0*L);
    vt_dot_p = -a_vm_p*vt_p;
    vm_dot_p = 0.0;

    f_p = [om_dot_p; vt_dot_p; vm_dot_p];
    F(:,i) = (f_p - f)/epsFD;
end

%% ---------- Q  ----------
vm_for_Q = max(vm, 0.1);
Q = zeros(3,3);
Q(1,1) = q_omega;
Q(2,2) = pi*(vm_for_Q^3)*(Ti^2)/L;
Q(3,3) = q_vm;

%% ---------- covariance prediction  ----------
Pdot   = F*P + P*F' + Q - (K_prev*Rm*K_prev');
P_pred = P + Ts*Pdot;

%% ---------- measurement update ----------
H = [1 0 0];
y = omega_r_meas;

innov = y - x_pred(1);
S = H*P_pred*H' + Rm;
K = (P_pred*H')/S;

x_upd = x_pred + K*innov;
P_upd = (eye(3) - K*H) * P_pred;

x_hat  = x_upd;
P      = P_upd;
K_prev = K;

%% ---------- outputs ----------
omega_r_hat = x_hat(1);
vt_hat      = x_hat(2);
vm_hat      = x_hat(3);
v_hat       = vt_hat + vm_hat;
end
